simulink model "Robot_control"  (Simulink 10.0)
settings: Solver=ode45  StartTime=0.0  StopTime=10  RelTol=1e-3
libraries: mblibv1 x4, simulink x2, vrlib x1
settings Model: Creator=zigg  LastModifiedBy=Vlad Petrenciuc
settings DataIOCC: SaveFormat=StructureWithTime
settings DebuggingCC: UnderspecifiedInitializationDetection=Simplified  MergeDetectMultiDrivingBlocksExec=error  FcnCallInpInsideContextMsg=warning  SFUnexpectedBacktrackingDiag=error  SFNoUnconditionalDefaultTransitionDiag=error
settings HardwareCC: ProdBitPerPointer=64  ProdLargestAtomicFloat=Float  ProdIntDivRoundTo=Zero  ProdEndianess=LittleEndian  ProdHWDeviceType=Specified
settings ModelReferenceCC: PropagateSignalLabelsOutOfModel=on
settings GRTTargetCC: TargetLangStandard=C99 (ISO)  CombineOutputUpdateFcns=on  GRTInterface=off
settings ConfigComp: CovMetricSettings=dwe  CovHtmlReporting=off  CovSaveCumulativeToWorkspaceVar=off  CovSaveSingleToWorkspaceVar=off

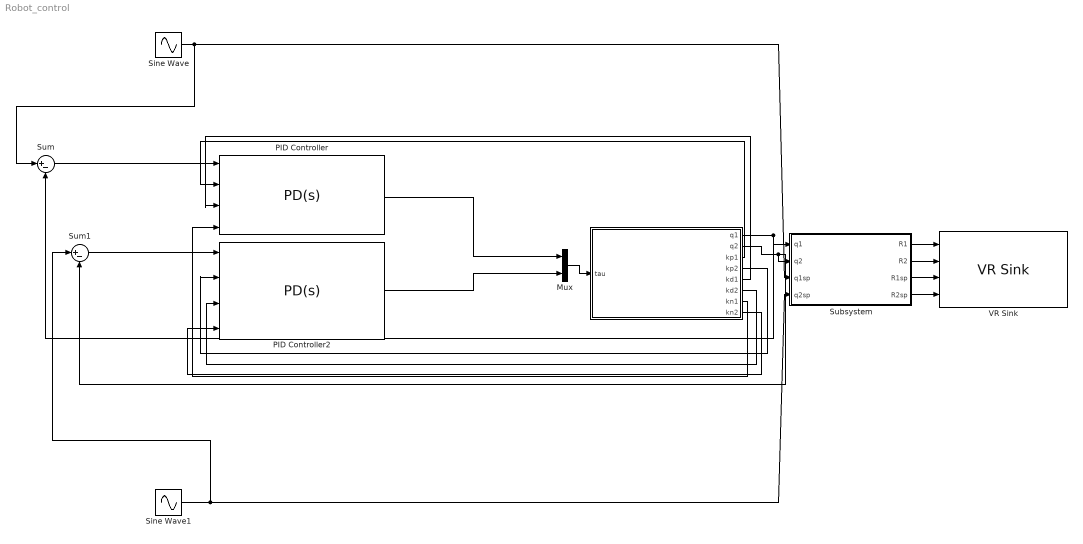
== system Robot_control ==
  "  " : Subsystem
  Mux : Mux  Inputs=2
  PID Controller : simulink/Continuous/PID Controller  Controller=PD  Form=Parallel  TimeDomain=Continuous-time  SampleTime=-1  IntegratorMethod=Forward Euler  FilterMethod=Forward Euler  ControllerParametersSource=external  P=1  I=1  D=0  UseFilter=on  N=100  TunerSelectOption=Transfer Function Based (PID Tuner App)  InitialConditionSource=internal  InitialConditionForIntegrator=0  InitialConditionForFilter=0  DifferentiatorICPrevScaledInput=0  ExternalReset=none  TrackingMode=off  Kt=1  LimitOutput=off  UpperSaturationLimit=inf  LowerSaturationLimit=-inf  LinearizeAsGain=on  AntiWindupMode=none  Kb=1  POutMin=[]  POutMax=[]  IOutMin=[]  IOutMax=[]  DOutMin=[]  DOutMax=[]  NOutMin=[]  NOutMax=[]  SumOutMin=[]  SumOutMax=[]  SaturationOutMin=[]  SaturationOutMax=[]  PParamMin=[]  PParamMax=[]  IParamMin=[]  IParamMax=[]  DParamMin=[]  DParamMax=[]  NParamMin=[]  NParamMax=[]  KbParamMin=[]  KbParamMax=[]  KtParamMin=[]  KtParamMax=[]  KbOutMin=[]  KbOutMax=[]  KtOutMin=[]  KtOutMax=[]  IntegratorOutMin=[]  IntegratorOutMax=[]  FilterOutMin=[]  FilterOutMax=[]  SumI1OutMin=[]  SumI1OutMax=[]  SumI2OutMin=[]  SumI2OutMax=[]  SumI3OutMin=[]  SumI3OutMax=[]  SumI4OutMin=[]  SumI4OutMax=[]  SumDOutMin=[]  SumDOutMax=[]  DifferentiatorOutMin=[]  DifferentiatorOutMax=[]  FilterDiffOutCoefMin=[]  FilterDiffOutCoefMax=[]  ReciprocalOutMin=[]  ReciprocalOutMax=[]  SumDenOutMin=[]  SumDenOutMax=[]  SumNumOutMin=[]  SumNumOutMax=[]  DivideOutMin=[]  DivideOutMax=[]  IntegratorContinuousStateAttributes=''  IntegratorStateMustResolveToSignalObject=off  IntegratorRTWStateStorageClass=Auto  FilterContinuousStateAttributes=''  FilterStateMustResolveToSignalObject=off  FilterRTWStateStorageClass=Auto  ParallelPVariant=ExternalParameters  IdealPVariant=Disabled  IVariant=Disabled  DVariant=ExternalParameters  IntegratorVariant=Disabled  SatVariant=Disabled  AWVariant=Disabled  PCopyVariant=Disabled  TRVariant=Disabled  FdbkBlocksVariant=Forward  IdealPFdbkVariant=Disabled  SatFdbkVariant=Disabled  DerivativeFilterVariant=ContFilter  NVariant=ExternalParameters  NCopyVariant=Disabled  FilterICVariant=InternalICsFilter  IntegratorICVariant=Disabled  ExternalResetVariant=Disabled  TRSumVariant=Passthrough  SumFdbkVariant=Disabled  SumVariant=Sum_PD
  PID Controller2 : simulink/Continuous/PID Controller  Controller=PD  Form=Parallel  TimeDomain=Continuous-time  SampleTime=-1  IntegratorMethod=Forward Euler  FilterMethod=Forward Euler  ControllerParametersSource=external  P=1  I=1  D=0  UseFilter=on  N=100  TunerSelectOption=Transfer Function Based (PID Tuner App)  InitialConditionSource=internal  InitialConditionForIntegrator=0  InitialConditionForFilter=0  DifferentiatorICPrevScaledInput=0  ExternalReset=none  TrackingMode=off  Kt=1  LimitOutput=off  UpperSaturationLimit=inf  LowerSaturationLimit=-inf  LinearizeAsGain=on  AntiWindupMode=none  Kb=1  POutMin=[]  POutMax=[]  IOutMin=[]  IOutMax=[]  DOutMin=[]  DOutMax=[]  NOutMin=[]  NOutMax=[]  SumOutMin=[]  SumOutMax=[]  SaturationOutMin=[]  SaturationOutMax=[]  PParamMin=[]  PParamMax=[]  IParamMin=[]  IParamMax=[]  DParamMin=[]  DParamMax=[]  NParamMin=[]  NParamMax=[]  KbParamMin=[]  KbParamMax=[]  KtParamMin=[]  KtParamMax=[]  KbOutMin=[]  KbOutMax=[]  KtOutMin=[]  KtOutMax=[]  IntegratorOutMin=[]  IntegratorOutMax=[]  FilterOutMin=[]  FilterOutMax=[]  SumI1OutMin=[]  SumI1OutMax=[]  SumI2OutMin=[]  SumI2OutMax=[]  SumI3OutMin=[]  SumI3OutMax=[]  SumI4OutMin=[]  SumI4OutMax=[]  SumDOutMin=[]  SumDOutMax=[]  DifferentiatorOutMin=[]  DifferentiatorOutMax=[]  FilterDiffOutCoefMin=[]  FilterDiffOutCoefMax=[]  ReciprocalOutMin=[]  ReciprocalOutMax=[]  SumDenOutMin=[]  SumDenOutMax=[]  SumNumOutMin=[]  SumNumOutMax=[]  DivideOutMin=[]  DivideOutMax=[]  IntegratorContinuousStateAttributes=''  IntegratorStateMustResolveToSignalObject=off  IntegratorRTWStateStorageClass=Auto  FilterContinuousStateAttributes=''  FilterStateMustResolveToSignalObject=off  FilterRTWStateStorageClass=Auto  ParallelPVariant=ExternalParameters  IdealPVariant=Disabled  IVariant=Disabled  DVariant=ExternalParameters  IntegratorVariant=Disabled  SatVariant=Disabled  AWVariant=Disabled  PCopyVariant=Disabled  TRVariant=Disabled  FdbkBlocksVariant=Forward  IdealPFdbkVariant=Disabled  SatFdbkVariant=Disabled  DerivativeFilterVariant=ContFilter  NVariant=ExternalParameters  NCopyVariant=Disabled  FilterICVariant=InternalICsFilter  IntegratorICVariant=Disabled  ExternalResetVariant=Disabled  TRSumVariant=Passthrough  SumFdbkVariant=Disabled  SumVariant=Sum_PD
  Sine Wave : Sin  SampleTime=0
  Sine Wave1 : Sin  SampleTime=0
  Subsystem : Subsystem
  Sum : Sum  Inputs=|+-
  Sum1 : Sum  Inputs=|+-
  VR Sink : vrlib/VR Sink  InstantiateOnLoad=on  SampleTime=0.1  ViewEnable=on  RemoteChange=off  RemoteView=off  FieldsWritten=Joint1.rotation.4.1.1.double#Joint2.rotation.4.1.1.double#Joint1_SP.rotation.4.1.1.double#Joint2_SP.rotation.4.1.1.double  WorldFileName=my_robot.wrl  AutoView=off  VideoDimensions=[]  AllowVariableSize=off
      settings: SourceProductName=Simulink
  wires:
  Subsystem/1(R1) -> VR Sink/1
  Subsystem/2(R2) -> VR Sink/2
  Subsystem/3(R1sp) -> VR Sink/3
  Subsystem/4(R2sp) -> VR Sink/4
  "  "/1(q1) -> Sum/2, Subsystem/1(q1)
  "  "/2(q2) -> Sum1/2, Subsystem/2(q2)
  Sine Wave1/1 -> Sum1/1, Subsystem/4(q2sp)
  Sine Wave/1 -> Sum/1, Subsystem/3(q1sp)
  Mux/1 -> "  "/1(tau)
  "  "/3(kp1) -> PID Controller/2
  "  "/5(kd1) -> PID Controller/3
  "  "/7(kn1) -> PID Controller/4
  PID Controller/1 -> Mux/1
  "  "/4(kp2) -> PID Controller2/2
  "  "/6(kd2) -> PID Controller2/3
  "  "/8(kn2) -> PID Controller2/4
  Sum/1 -> PID Controller/1
  Sum1/1 -> PID Controller2/1
  PID Controller2/1 -> Mux/2

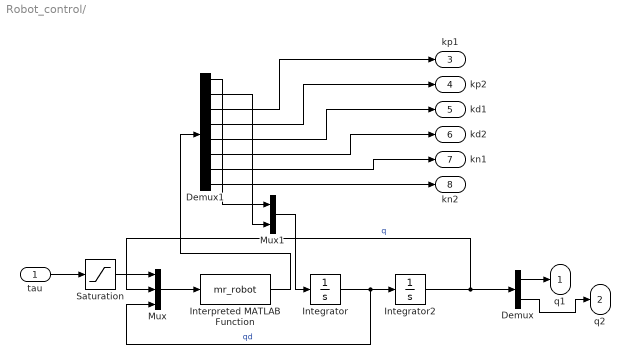
== system Robot_control/   ==
  tau : Inport
  Demux : Demux  Outputs=2
  Demux1 : Demux  Outputs=8
  Integrator : Integrator
  Integrator2 : Integrator  InitialCondition=pi/2*0
  Interpreted MATLAB Function : MATLABFcn  MATLABFcn=mr_robot  OutputDimensions=8
  Mux : Mux  Inputs=3
  Mux1 : Mux  Inputs=2
  Saturation : Saturate  UpperLimit=1.18  LowerLimit=-1.18
  q1 : Outport
  q2 : Outport  Port=2
  kp1 : Outport  Port=3
  kp2 : Outport  Port=4
  kd1 : Outport  Port=5
  kd2 : Outport  Port=6
  kn1 : Outport  Port=7
  kn2 : Outport  Port=8
  wires:
  Interpreted MATLAB Function/1 -> Demux1/1
  Integrator2/1 -> Demux/1, Mux/2  "q"
  Integrator/1 -> Mux/3, Integrator2/1  "qd"
  tau/1 -> Saturation/1
  Mux/1 -> Interpreted MATLAB Function/1
  Demux/1 -> q1/1
  Demux/2 -> q2/1
  Saturation/1 -> Mux/1
  Demux1/3 -> kp1/1
  Demux1/4 -> kp2/1
  Demux1/5 -> kd1/1
  Demux1/6 -> kd2/1
  Demux1/7 -> kn1/1
  Demux1/8 -> kn2/1
  Demux1/1 -> Mux1/1
  Demux1/2 -> Mux1/2
  Mux1/1 -> Integrator/1

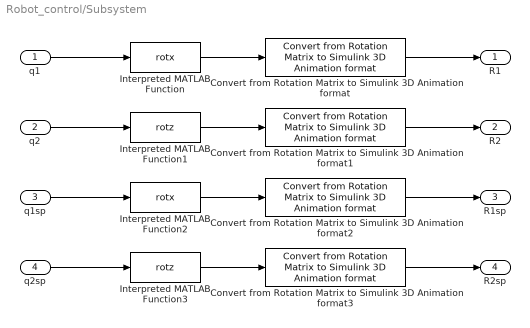
== system Robot_control/Subsystem ==
  q1 : Inport
  q2 : Inport  Port=2
  q1sp : Inport  Port=3
  q2sp : Inport  Port=4
  Convert from Rotation Matrix to Simulink 3D Animation format{,1..3} (4 alike) : mblibv1/Utilities/Convert from Rotation Matrix to Simulink 3D Animation format
      settings: SourceProductName=Simscape Multibody  SourceProductBaseCode=MS
  Interpreted MATLAB Function : MATLABFcn  MATLABFcn=rotx
  Interpreted MATLAB Function1 : MATLABFcn  MATLABFcn=rotz
  Interpreted MATLAB Function2 : MATLABFcn  MATLABFcn=rotx
  Interpreted MATLAB Function3 : MATLABFcn  MATLABFcn=rotz
  R1 : Outport
  R2 : Outport  Port=2
  R1sp : Outport  Port=3
  R2sp : Outport  Port=4
  wires:
  Convert from Rotation Matrix to Simulink 3D Animation format/1 -> R1/1
  Interpreted MATLAB Function/1 -> Convert from Rotation Matrix to Simulink 3D Animation format/1
  Interpreted MATLAB Function1/1 -> Convert from Rotation Matrix to Simulink 3D Animation format1/1
  Interpreted MATLAB Function2/1 -> Convert from Rotation Matrix to Simulink 3D Animation format2/1
  Interpreted MATLAB Function3/1 -> Convert from Rotation Matrix to Simulink 3D Animation format3/1
  q1/1 -> Interpreted MATLAB Function/1
  q2/1 -> Interpreted MATLAB Function1/1
  q1sp/1 -> Interpreted MATLAB Function2/1
  q2sp/1 -> Interpreted MATLAB Function3/1
  Convert from Rotation Matrix to Simulink 3D Animation format1/1 -> R2/1
  Convert from Rotation Matrix to Simulink 3D Animation format2/1 -> R1sp/1
  Convert from Rotation Matrix to Simulink 3D Animation format3/1 -> R2sp/1
